simulink model "less_conservative_FBA"  (R2015b)
settings: Solver=VariableStepAuto  StartTime=0.0  StopTime=20  RelTol=1e-3
values from neighbouring files (symbols this model uses):
  bHI = 0    [Initiation.m]
  bWall = block.DialogPrm(2).Data    [HapticController.m]    (also in Initiation.m = 0; VirtualEnvironment5.m)
  dof = block.DialogPrm(2).Data    [Controller.m]    (also in Controller1.m; Controller_more.m = block.DialogPrm(3).Data; Initiation.m = 1; Parameters.m = 1)
  kWall = block.DialogPrm(1).Data    [HapticController.m]    (also in Initiation.m = 5000; VirtualEnvironment5.m)
  m = 1    [Initiation.m]
  mu = 0    [Controller1.m]
  nWall = block.DialogPrm(6).Data    [Controller1.m]    (also in HapticController.m = block.DialogPrm(3).Data; Initial_Conditions.m = -1; Initiation.m = -1; MoreConservative.m = block.DialogPrm(5).Data)
  p0 = block.DialogPrm(4).Data    [Controller.m]    (also in Controller1.m; Initiation.m = 0.12; Parameters.m = 1; VirtualEnvironment.m = block.DialogPrm(8).Data)
  tsampling = block.DialogPrm(3).Data    [Controller.m]    (also in Controller1.m; Controller_more.m = block.DialogPrm(4).Data; HapticController.m = block.DialogPrm(6).Data; Initial_Conditions.m = 0.001)
  v0 = block.DialogPrm(6).Data    [HapticDevice.m]    (also in HumanOperator.m; Initiation.m = 0; Parameters.m = 0; VirtualEnvironment4.m = block.DialogPrm(8).Data)
  xWall = 0.126    [Initiation.m]    (also in MoreConservative.m = block.DialogPrm(4).Data; Parameters.m = [1 2 3 4 5 6 7 8]*0.0005; VirtualEnvironment.m = block.DialogPrm(3).Data; VirtualEnvironment5.m = block.DialogPrm(4).Data)
libraries: simulink x2
settings Model: Creator=TOSHIBA  LastModifiedBy=TOSHIBA

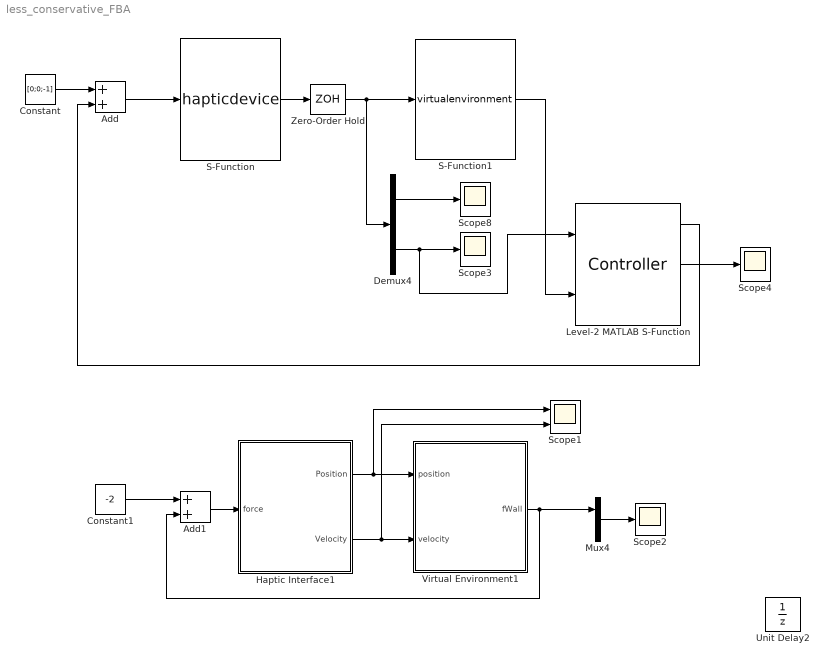
== system less_conservative_FBA ==
  Add : Sum
  Add1 : Sum
  Constant : Constant  Value=[0;0;-1]
  Constant1 : Constant  Value=-2
  Demux4 : Demux  Outputs=2
  Haptic Interface1 : Subsystem
  Level-2 MATLAB S-Function : M-S-Function  FunctionName=Controller  Parameters=bHI,dof,tsampling,p0
  Mux4 : Mux  Inputs=2
  S-Function : S-Function  FunctionName=hapticdevice  Parameters=m,bHI,v0,p0  SFunctionDeploymentMode=off  EnableBusSupport=off
  S-Function1 : S-Function  FunctionName=virtualenvironment  Parameters=kWall,bWall,xWall,[0;0;0],mu  SFunctionDeploymentMode=off  EnableBusSupport=off
  Scope1 : Scope  NumInputPorts=2
  Scope{2..4,8} (4 alike) : Scope
  Unit Delay2 : UnitDelay  InitialCondition=[0;0;0]  SampleTime=tsampling
  Virtual Environment1 : Subsystem
  Zero-Order Hold : ZeroOrderHold  SampleTime=tsampling
  wires:
  Constant/1 -> Add/1
  Haptic Interface1/2(Velocity) -> Scope1/2, Virtual Environment1/2(velocity)
  Haptic Interface1/1(Position) -> Scope1/1, Virtual Environment1/1(position)
  Add1/1 -> Haptic Interface1/1(force)
  Constant1/1 -> Add1/1
  Virtual Environment1/1(fWall) -> Mux4/1, Add1/2
  Zero-Order Hold/1 -> S-Function1/1, Demux4/1
  Demux4/2 -> Level-2 MATLAB S-Function/1, Scope3/1
  Demux4/1 -> Scope8/1
  Mux4/1 -> Scope2/1
  Level-2 MATLAB S-Function/2 -> Scope4/1
  Add/1 -> S-Function/1
  S-Function/1 -> Zero-Order Hold/1
  Level-2 MATLAB S-Function/1 -> Add/2
  S-Function1/1 -> Level-2 MATLAB S-Function/2

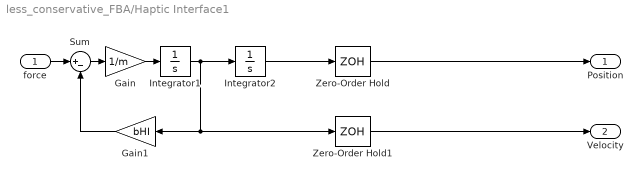
== system less_conservative_FBA/Haptic Interface1 ==
  force : Inport
  Gain : Gain  Gain=1/m
  Gain1 : Gain  Gain=bHI
  Integrator1 : Integrator  InitialCondition=v0(1)
  Integrator2 : Integrator  InitialCondition=p0(3)
  Sum : Sum  Inputs=|+-
  Zero-Order Hold : ZeroOrderHold  SampleTime=tsampling
  Zero-Order Hold1 : ZeroOrderHold  SampleTime=tsampling
  Position : Outport
  Velocity : Outport  Port=2
  wires:
  Integrator1/1 -> Zero-Order Hold1/1, Gain1/1, Integrator2/1
  Sum/1 -> Gain/1
  force/1 -> Sum/1
  Gain/1 -> Integrator1/1
  Gain1/1 -> Sum/2
  Integrator2/1 -> Zero-Order Hold/1
  Zero-Order Hold/1 -> Position/1
  Zero-Order Hold1/1 -> Velocity/1

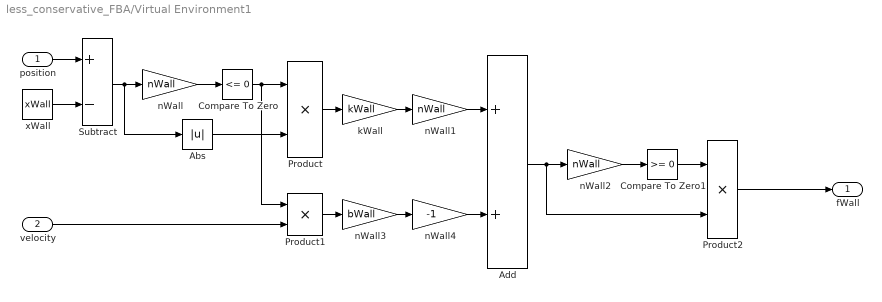
== system less_conservative_FBA/Virtual Environment1 ==
  position : Inport
  velocity : Inport  Port=2
  Abs : Abs
  Add : Sum
  Compare To Zero : simulink/Logic and Bit Operations/Compare To Zero  relop=<=  OutDataTypeStr=boolean
  Compare To Zero1 : simulink/Logic and Bit Operations/Compare To Zero  relop=>=  OutDataTypeStr=boolean
  Product : Product
  Product1 : Product
  Product2 : Product
  Subtract : Sum  Inputs=+-
  kWall : Gain  Gain=kWall
  nWall : Gain  Gain=nWall
  nWall1 : Gain  Gain=nWall
  nWall2 : Gain  Gain=nWall
  nWall3 : Gain  Gain=bWall
  nWall4 : Gain  Gain=-1
  xWall : Constant  Value=xWall
  fWall : Outport
  wires:
  Compare To Zero1/1 -> Product2/1
  nWall2/1 -> Compare To Zero1/1
  kWall/1 -> nWall1/1
  Product/1 -> kWall/1
  Abs/1 -> Product/2
  Compare To Zero/1 -> Product1/1, Product/1
  nWall/1 -> Compare To Zero/1
  Subtract/1 -> nWall/1, Abs/1
  position/1 -> Subtract/1
  xWall/1 -> Subtract/2
  nWall3/1 -> nWall4/1
  Product1/1 -> nWall3/1
  velocity/1 -> Product1/2
  nWall1/1 -> Add/1
  nWall4/1 -> Add/2
  Add/1 -> Product2/2, nWall2/1
  Product2/1 -> fWall/1
